simulink model "Longitudinal_Simulink"  (Simulink 7.1)
settings: Solver=ode45  StartTime=0.0  StopTime=1.0  RelTol=1e-3
settings Model: Creator=Meisel  LastModifiedBy=Meisel

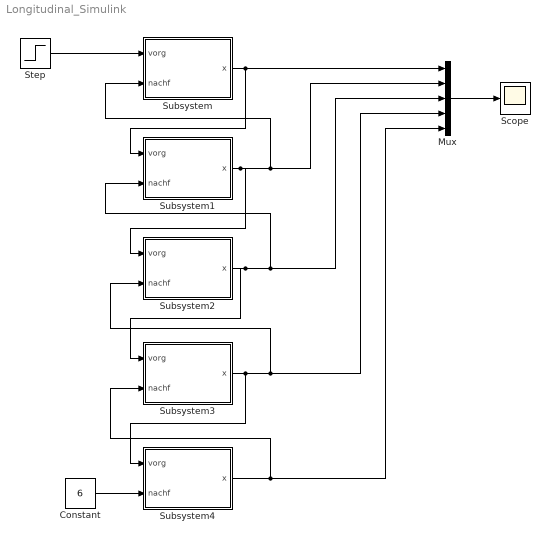
== system Longitudinal_Simulink ==
  Constant : Constant  Value=6  OutDataType=sfix(16)  OutScaling=2^0
  Mux : Mux  Inputs=5
  Scope : Scope
  Step : Step  Time=0.1  After=0.5  SampleTime=0
  Subsystem : Subsystem  mask{Integrator=1111}
      mask prompts: Integrator "Initial"
  Subsystem1 : Subsystem
  Subsystem2 : Subsystem
  Subsystem3 : Subsystem
  Subsystem4 : Subsystem
  wires:
  Subsystem/1(x) -> Subsystem1/1(vorg), Mux/1
  Subsystem2/1(x) -> Subsystem3/1(vorg), Subsystem1/2(nachf), Mux/3
  Subsystem1/1(x) -> Subsystem2/1(vorg), Subsystem/2(nachf), Mux/2
  Subsystem3/1(x) -> Subsystem2/2(nachf), Mux/4, Subsystem4/1(vorg)
  Step/1 -> Subsystem/1(vorg)
  Mux/1 -> Scope/1
  Constant/1 -> Subsystem4/2(nachf)
  Subsystem4/1(x) -> Mux/5, Subsystem3/2(nachf)

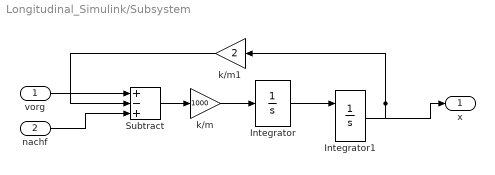
== system Longitudinal_Simulink/Subsystem ==
  vorg : Inport  OutDataType=sfix(16)  OutScaling=2^0
  nachf : Inport  Port=2  OutDataType=sfix(16)  OutScaling=2^0
  Integrator : Integrator
  Integrator1 : Integrator  InitialConditionSource=external  InitialCondition=1
  Subtract : Sum  Inputs=+-+  OutDataType=sfix(16)  OutScaling=2^-10
  k/m : Gain  Gain=1000  ParameterDataType=sfix(16)  ParameterScaling=2^0  OutDataType=sfix(16)  OutScaling=2^0
  k/m1 : Gain  Orientation=left  Gain=2  ParameterDataType=sfix(16)  ParameterScaling=2^0  OutDataType=sfix(16)  OutScaling=2^0
  x : Outport  OutDataType=sfix(16)  OutScaling=2^0
  wires:
  Integrator/1 -> Integrator1/1
  Subtract/1 -> k/m/1
  k/m/1 -> Integrator/1
  Integrator1/1 -> x/1, k/m1/1
  nachf/1 -> Subtract/3
  vorg/1 -> Subtract/1
  k/m1/1 -> Subtract/2

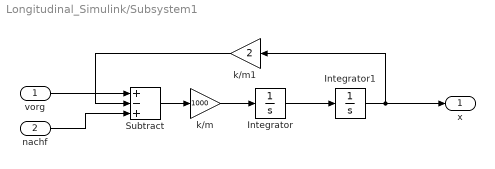
== system Longitudinal_Simulink/Subsystem1 ==
  vorg : Inport  OutDataType=sfix(16)  OutScaling=2^0
  nachf : Inport  Port=2  OutDataType=sfix(16)  OutScaling=2^0
  Integrator : Integrator
  Integrator1 : Integrator  InitialCondition=2
  Subtract : Sum  Inputs=+-+  OutDataType=sfix(16)  OutScaling=2^-10
  k/m : Gain  Gain=1000  ParameterDataType=sfix(16)  ParameterScaling=2^0  OutDataType=sfix(16)  OutScaling=2^0
  k/m1 : Gain  Orientation=left  Gain=2  ParameterDataType=sfix(16)  ParameterScaling=2^0  OutDataType=sfix(16)  OutScaling=2^0
  x : Outport  OutDataType=sfix(16)  OutScaling=2^0
  wires:
  Integrator/1 -> Integrator1/1
  Subtract/1 -> k/m/1
  k/m/1 -> Integrator/1
  Integrator1/1 -> x/1, k/m1/1
  nachf/1 -> Subtract/3
  vorg/1 -> Subtract/1
  k/m1/1 -> Subtract/2

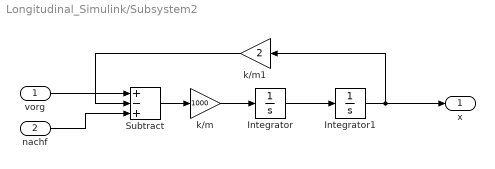
== system Longitudinal_Simulink/Subsystem2 ==
  vorg : Inport  OutDataType=sfix(16)  OutScaling=2^0
  nachf : Inport  Port=2  OutDataType=sfix(16)  OutScaling=2^0
  Integrator : Integrator
  Integrator1 : Integrator  InitialCondition=3
  Subtract : Sum  Inputs=+-+  OutDataType=sfix(16)  OutScaling=2^-10
  k/m : Gain  Gain=1000  ParameterDataType=sfix(16)  ParameterScaling=2^0  OutDataType=sfix(16)  OutScaling=2^0
  k/m1 : Gain  Orientation=left  Gain=2  ParameterDataType=sfix(16)  ParameterScaling=2^0  OutDataType=sfix(16)  OutScaling=2^0
  x : Outport  OutDataType=sfix(16)  OutScaling=2^0
  wires:
  Integrator/1 -> Integrator1/1
  Subtract/1 -> k/m/1
  k/m/1 -> Integrator/1
  Integrator1/1 -> x/1, k/m1/1
  nachf/1 -> Subtract/3
  vorg/1 -> Subtract/1
  k/m1/1 -> Subtract/2

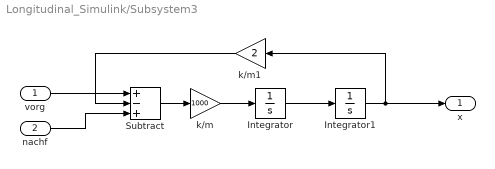
== system Longitudinal_Simulink/Subsystem3 ==
  vorg : Inport  OutDataType=sfix(16)  OutScaling=2^0
  nachf : Inport  Port=2  OutDataType=sfix(16)  OutScaling=2^0
  Integrator : Integrator
  Integrator1 : Integrator  InitialCondition=4
  Subtract : Sum  Inputs=+-+  OutDataType=sfix(16)  OutScaling=2^-10
  k/m : Gain  Gain=1000  ParameterDataType=sfix(16)  ParameterScaling=2^0  OutDataType=sfix(16)  OutScaling=2^0
  k/m1 : Gain  Orientation=left  Gain=2  ParameterDataType=sfix(16)  ParameterScaling=2^0  OutDataType=sfix(16)  OutScaling=2^0
  x : Outport  OutDataType=sfix(16)  OutScaling=2^0
  wires:
  Integrator/1 -> Integrator1/1
  Subtract/1 -> k/m/1
  k/m/1 -> Integrator/1
  Integrator1/1 -> x/1, k/m1/1
  nachf/1 -> Subtract/3
  vorg/1 -> Subtract/1
  k/m1/1 -> Subtract/2

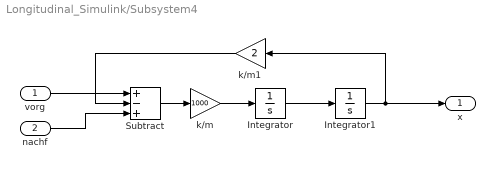
== system Longitudinal_Simulink/Subsystem4 ==
  vorg : Inport  OutDataType=sfix(16)  OutScaling=2^0
  nachf : Inport  Port=2  OutDataType=sfix(16)  OutScaling=2^0
  Integrator : Integrator
  Integrator1 : Integrator  InitialCondition=5
  Subtract : Sum  Inputs=+-+  OutDataType=sfix(16)  OutScaling=2^-10
  k/m : Gain  Gain=1000  ParameterDataType=sfix(16)  ParameterScaling=2^0  OutDataType=sfix(16)  OutScaling=2^0
  k/m1 : Gain  Orientation=left  Gain=2  ParameterDataType=sfix(16)  ParameterScaling=2^0  OutDataType=sfix(16)  OutScaling=2^0
  x : Outport  OutDataType=sfix(16)  OutScaling=2^0
  wires:
  Integrator/1 -> Integrator1/1
  Subtract/1 -> k/m/1
  k/m/1 -> Integrator/1
  Integrator1/1 -> x/1, k/m1/1
  nachf/1 -> Subtract/3
  vorg/1 -> Subtract/1
  k/m1/1 -> Subtract/2
